simulink model "blockdemo_complex"  (Simulink 7.6)
settings: Solver=ode45  StartTime=0.0  StopTime=100.0  RelTol=1e-3
InitFcn:
  | %% DSPBuilder Start
  | alt_dspbuilder_update_model(bdroot)
  | %% DSPBuilder End
libraries: allblocks_alteradspbuilder2 x8
settings Model: Creator=akarapet  LastModifiedBy=akarapet

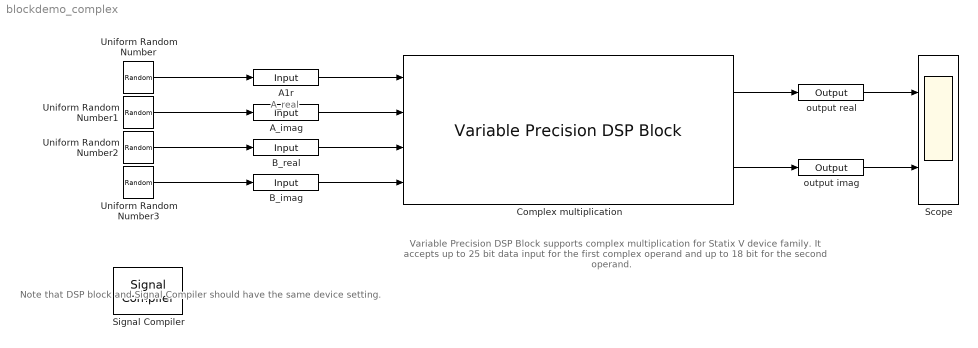
== system blockdemo_complex ==
  note: A_real
  note: Variable Precision DSP Block supports complex
      | multiplication for Statix V device family.
      | It accepts up to 25 bit data input for the first complex
      | operand and up to 18 bit  for the second operand.
  note: Note that DSP block and Signal Compiler
      | should have the same device setting.
  A1r : allblocks_alteradspbuilder2/Input  iofile=/data/akarapet/qshell_linux64_regtests/p4/dsp_builder/dsp_builder2/Documentation/DesignExamples/Tutorials/UnitBlocks/Arithmetic/VariablePrecisionDSPBlock/tb_blockdemo_complex/blockdemo%5Fcomplex_A1r.salt  BusType=Signed Integer  bwl=25  bwr=2  SpecifyClock=off  clock=default_clock  PORTTYPE=Input  externalType=Inferred  allowFloatingPointOverride=on  logOutputs=off
  A_imag : allblocks_alteradspbuilder2/Input  iofile=/data/akarapet/qshell_linux64_regtests/p4/dsp_builder/dsp_builder2/Documentation/DesignExamples/Tutorials/UnitBlocks/Arithmetic/VariablePrecisionDSPBlock/tb_blockdemo_complex/blockdemo%5Fcomplex_A%5Fimag.salt  BusType=Signed Integer  bwl=25  bwr=2  SpecifyClock=off  clock=default_clock  PORTTYPE=Input  externalType=Inferred  allowFloatingPointOverride=on  logOutputs=off
  B_imag : allblocks_alteradspbuilder2/Input  iofile=/data/akarapet/qshell_linux64_regtests/p4/dsp_builder/dsp_builder2/Documentation/DesignExamples/Tutorials/UnitBlocks/Arithmetic/VariablePrecisionDSPBlock/tb_blockdemo_complex/blockdemo%5Fcomplex_B%5Fimag.salt  BusType=Signed Integer  bwl=18  bwr=2  SpecifyClock=off  clock=default_clock  PORTTYPE=Input  externalType=Inferred  allowFloatingPointOverride=on  logOutputs=off
  B_real : allblocks_alteradspbuilder2/Input  iofile=/data/akarapet/qshell_linux64_regtests/p4/dsp_builder/dsp_builder2/Documentation/DesignExamples/Tutorials/UnitBlocks/Arithmetic/VariablePrecisionDSPBlock/tb_blockdemo_complex/blockdemo%5Fcomplex_B%5Freal.salt  BusType=Signed Integer  bwl=18  bwr=2  SpecifyClock=off  clock=default_clock  PORTTYPE=Input  externalType=Inferred  allowFloatingPointOverride=on  logOutputs=off
  Complex multiplication : allblocks_alteradspbuilder2/Variable Precision DSP Block  complex_model_delayed=0  model_delayed=0  device_family=Stratix V  used_mode_stratix=25x18 Complex Mode  used_mode_arria=Other Modes  in_25x18_complex_mode=1  in_18x18plus36_mode=0  in_other_modes=0  number_of_mults=1  clock_ena_inputs=off  async_clear_inputs=off  bus_type=Signed Integer  bwl_A=8  bwr_A=0  width_A=8  chain_width=64  reg_inputs_A=on  A_inputs_reg_ena=ENABLE 0  bwl_B=8  bwr_B=0  width_B=8  reg_inputs_B=on  B_inputs_reg_ena=ENABLE 0  bwl_joint_A_B=8  bwr_joint_A_B=0  reg_joint_A_B_input=on  A_B_input_reg_ena=ENABLE 0  bwl_A_complex=25  bwr_A_complex=2  reg_complex_A=off  A_complex_inputs_reg_ena=ENABLE 0  bwl_B_complex=18  bwr_B_complex=2  reg_complex_B=off  B_complex_inputs_reg_ena=ENABLE 0  A_inputs_exist=1  B_inputs_exist=1  C_inputs_exist=0  coef_sel_inputs_exist=0  all_inputs_registered=0  no_input_registered=0  all_inputs_share_same_clocks=0  full_resolution=off  bwl_out=44  bwr_out=2  reg_output=off  output_reg_ena=ENABLE 0  systolic_regs_available=0  enable_systolic_regs=off  systolic_regs_used=0  basic_struct_ok_for_input_scan=0  input_scan_available=0  enable_input_scan=off  input_scan_used=0  input_scan_delay_regs_available=0  enable_input_scan_delay_regs=off  input_scan_delay_regs_used=0  basic_struct_ok_for_coef_rom=0  coef_rom_available=0  enable_coef_rom=off  coef_rom_used=0  basic_struct_ok_for_preadder=0  preadder_available=0  enable_preadder=off  preadder_used=0  preadder_direction=ADD  square_mode_available=0  enable_square_mode=off  square_mode_used=0  upper_limit_9bit=9  upper_limit_18bit=18  upper_limit_27bit=27  in_18x18_modes=0  in_27x27_modes=0  in_36x18_modes=0  in_36x36_mode=0  mult1_adder_available=0  mult1_direction=ADD  mult3_adder_available=0  mult3_direction=ADD  chainout_adder_available=0  use_chainout_input=off  chainout_input_used=0  use_chainout_output=off  chainout_output_used=0  accum_available=0  enable_accum=off  accum_used=0  double_accum_available=0  enable_double_accum=off  double_accum_used=0  negate_available=0  mult_add_operation=ADD  rounding_constant_available=0  use_rounding_constant=off  rounding_constant_used=0  constant_value=1  bwl_C=8  bwr_C=0  bwl_coef=18  bwr_coef=0  mult0_coeffs=[0, 0, 0, 0, 0, 0, 0, 0]  mult1_coeffs=[0, 0, 0, 0, 0, 0, 0, 0]  mult2_coeffs=[0, 0, 0, 0, 0, 0, 0, 0]  mult3_coeffs=[0, 0, 0, 0, 0, 0, 0, 0]  reg_mult1_op_control=off  reg_mult3_op_control=off  reg_accum_control=off  reg_negate_control=off  control_regs_ena=ENABLE 0
  Scope : Scope  NumInputPorts=2
      settings: YMin=-5~-5  YMax=5~5
  Signal Compiler : allblocks_alteradspbuilder2/Signal Compiler  DeviceFamily=Stratix V  DeviceName=AUTO  EnableSignalTap=off  SignalTapDepth=128  UseBoardBlock=off  StpUseDefaultClock=on  StpClock=Clock  ExportDir=<binary blob, 153 chars, not shown>
  Uniform Random Number : UniformRandomNumber  Minimum=-78765654  Maximum=676567654  Seed=1591  SampleTime=1
  Uniform Random Number1 : UniformRandomNumber  Minimum=-98987654  Maximum=77765676  Seed=2365  SampleTime=1
  Uniform Random Number2 : UniformRandomNumber  Minimum=-98785432  Maximum=555565556  Seed=8888  SampleTime=1
  Uniform Random Number3 : UniformRandomNumber  Minimum=-878987  Maximum=7655556765  Seed=6657  SampleTime=1
  output imag : allblocks_alteradspbuilder2/Output  iofile=/data/akarapet/qshell_linux64_regtests/p4/dsp_builder/dsp_builder2/Documentation/DesignExamples/Tutorials/UnitBlocks/Arithmetic/VariablePrecisionDSPBlock/tb_blockdemo_complex/blockdemo%5Fcomplex_output+imag.capture  BusType=Signed Integer  bwl=44  bwr=0  externalType=Inferred  PORTTYPE=Output  allowFloatingPointOverride=on  logOutputs=off
  output real : allblocks_alteradspbuilder2/Output  iofile=/data/akarapet/qshell_linux64_regtests/p4/dsp_builder/dsp_builder2/Documentation/DesignExamples/Tutorials/UnitBlocks/Arithmetic/VariablePrecisionDSPBlock/tb_blockdemo_complex/blockdemo%5Fcomplex_output+real.capture  BusType=Signed Integer  bwl=44  bwr=0  externalType=Inferred  PORTTYPE=Output  allowFloatingPointOverride=on  logOutputs=off
  wires:
  Uniform Random Number/1 -> A1r/1
  Uniform Random Number1/1 -> A_imag/1
  Uniform Random Number2/1 -> B_real/1
  Uniform Random Number3/1 -> B_imag/1
  A1r/1 -> Complex multiplication/1
  A_imag/1 -> Complex multiplication/2
  B_real/1 -> Complex multiplication/3
  B_imag/1 -> Complex multiplication/4
  Complex multiplication/1 -> output real/1
  Complex multiplication/2 -> output imag/1
  output real/1 -> Scope/1
  output imag/1 -> Scope/2
